simulink model "two_blocks_w_spring"  (R2017a)
settings: Solver=VariableStepAuto  StartTime=0.0  StopTime=40  RelTol=1e-3
values from neighbouring files (symbols this model uses):
  a = 20    [two_block_spring.mat]
  d_e = 0.5    [animation_two_block_spring.m]    (also in two_block_spring.mat)
  e_h = -1    [animation_two_block_spring.m]    (also in two_block_spring.mat = 1)
  e_v = -1    [animation_two_block_spring.m]    (also in two_block_spring.mat = 1)
  g = 9.81    [two_block_spring.mat]
  k = 5    [two_block_spring.mat]
  m_h = [-w_h w_h w_h -w_h -w_h ; w_h w_h -w_h -w_h w_h]    [animation_two_block_spring.m]    (also in two_block_spring.mat = 1)
  m_v = [-w_v w_v w_v -w_v -w_v ; w_v w_v -w_v -w_v w_v]    [animation_two_block_spring.m]    (also in two_block_spring.mat = 0.5)
  mu_h = 0.1    [two_block_spring.mat]
  mu_v = 0.2    [two_block_spring.mat]
settings Model: Creator=Sorawit Inprom  LastModifiedBy=Sorawit Inprom

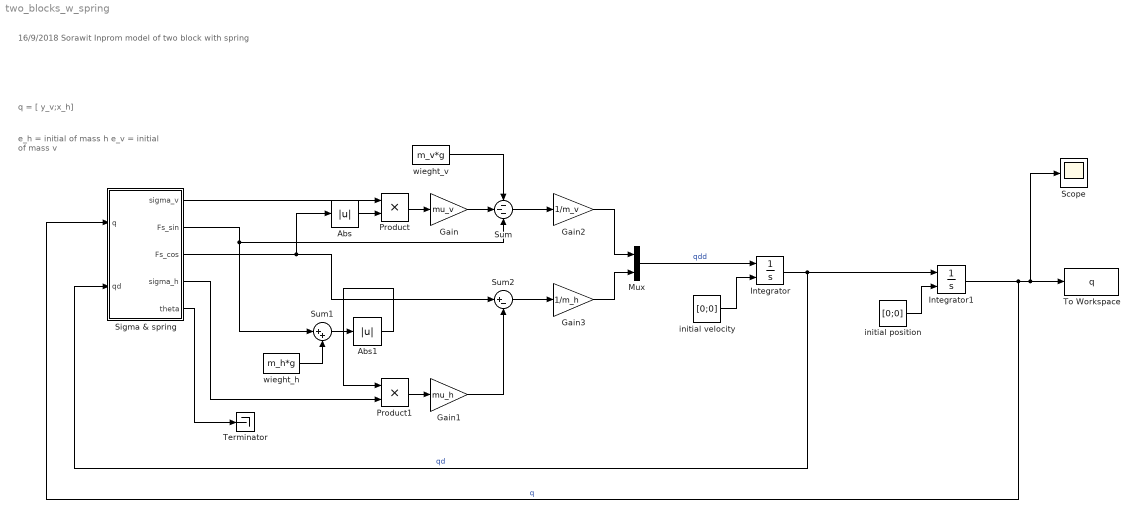
== system two_blocks_w_spring ==
  note: 16/9/2018
      | Sorawit Inprom
      | model of two block with spring
  note: e_h = initial of mass h
      | e_v = initial of mass v
  note: q = [ y_v;x_h]
  Abs : Abs
  Abs1 : Abs
  Gain : Gain  Gain=mu_v
  Gain1 : Gain  Gain=mu_h
  Gain2 : Gain  Gain=1/m_v
  Gain3 : Gain  Gain=1/m_h
  Integrator : Integrator  InitialConditionSource=external  InitialCondition=[0;0]  ContinuousStateAttributes='velocity'
  Integrator1 : Integrator  InitialConditionSource=external  InitialCondition=[e_v;e_h]  ContinuousStateAttributes='position'
  Mux : Mux  Inputs=2
  Product : Product
  Product1 : Product
  Scope : Scope
  Sigma & spring : Subsystem
  Sum : Sum  Inputs=---
  Sum1 : Sum  Inputs=|++
  Sum2 : Sum  Inputs=|+-
  Terminator : Terminator
  To Workspace : ToWorkspace  VariableName=q  SaveFormat=Timeseries  SampleTime=-1
  initial position : Constant  Value=[0;0]
  initial velocity : Constant  Value=[0;0]
  wieght_h : Constant  Value=m_h*g
  wieght_v : Constant  Value=m_v*g
  wires:
  Integrator/1 -> Sigma & spring/2(qd), Integrator1/1  "qd"
  Mux/1 -> Integrator/1  "qdd"
  wieght_v/1 -> Sum/1
  Product/1 -> Gain/1
  Product1/1 -> Gain1/1
  Gain1/1 -> Sum2/2
  Gain/1 -> Sum/2
  wieght_h/1 -> Sum1/2
  Sum/1 -> Gain2/1
  Sum2/1 -> Gain3/1
  Gain2/1 -> Mux/1
  Gain3/1 -> Mux/2
  initial velocity/1 -> Integrator/2
  initial position/1 -> Integrator1/2
  Integrator1/1 -> Sigma & spring/1(q), Scope/1, To Workspace/1  "q"
  Sigma & spring/1(sigma_v) -> Product/1
  Sigma & spring/3(Fs_cos) -> Abs/1, Sum2/1
  Sigma & spring/2(Fs_sin) -> Sum1/1, Sum/3
  Sigma & spring/4(sigma_h) -> Product1/2
  Sigma & spring/5("theta ") -> Terminator/1
  Abs/1 -> Product/2
  Sum1/1 -> Abs1/1
  Abs1/1 -> Product1/1

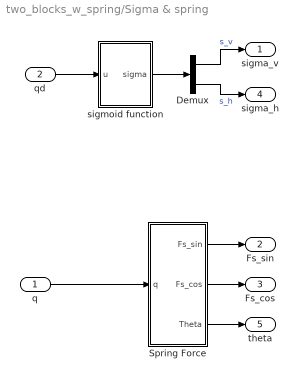
== system two_blocks_w_spring/Sigma & spring ==
  q : Inport
  qd : Inport  Port=2
  Demux : Demux  Outputs=2
  Spring Force : Subsystem
  sigmoid function : Subsystem
  sigma_v : Outport
  Fs_sin : Outport  Port=2
  Fs_cos : Outport  Port=3
  sigma_h : Outport  Port=4
  "theta " : Outport  Port=5
  wires:
  Demux/1 -> sigma_v/1  "s_v"
  q/1 -> Spring Force/1(q)
  sigmoid function/1(sigma) -> Demux/1
  Spring Force/1(Fs_sin) -> Fs_sin/1
  Spring Force/2(Fs_cos) -> Fs_cos/1
  qd/1 -> sigmoid function/1(u)
  Demux/2 -> sigma_h/1  "s_h"
  Spring Force/3(Theta) -> "theta "/1

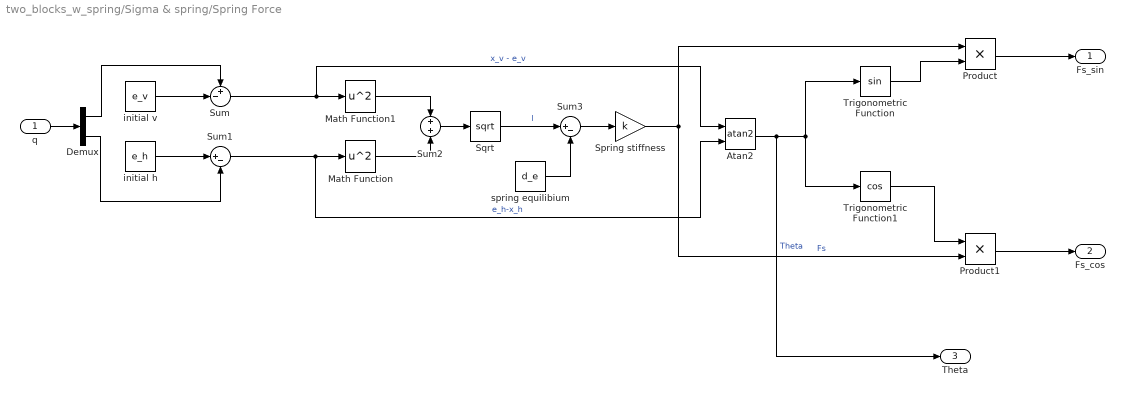
== system two_blocks_w_spring/Sigma & spring/Spring Force ==
  q : Inport
  Atan2 : Trigonometry  Operator=atan2
  Demux : Demux  Outputs=2
  Math Function : Math  Operator=square  SaturateOnIntegerOverflow=on
  Math Function1 : Math  Operator=square  SaturateOnIntegerOverflow=on
  Product : Product
  Product1 : Product
  Spring stiffness : Gain  Gain=k
  Sqrt : Sqrt  SaturateOnIntegerOverflow=on
  Sum : Sum  Inputs=+-|
  Sum1 : Sum  Inputs=|+-
  Sum2 : Sum  Inputs=+|+
  Sum3 : Sum  Inputs=|+-
  Trigonometric Function : Trigonometry
  Trigonometric Function1 : Trigonometry  Operator=cos
  initial h : Constant  Value=e_h
  initial v : Constant  Value=e_v
  spring equilibium : Constant  Value=d_e
  Fs_sin : Outport
  Fs_cos : Outport  Port=2
  Theta : Outport  Port=3
  wires:
  initial v/1 -> Sum/2
  Sqrt/1 -> Sum3/1  "l"
  Atan2/1 -> Theta/1, Trigonometric Function1/1, Trigonometric Function/1  "Theta"
  initial h/1 -> Sum1/1
  Sum1/1 -> Math Function/1, Atan2/2  "e_h-x_h"
  q/1 -> Demux/1
  Sum/1 -> Math Function1/1, Atan2/1  "x_v - e_v"
  Demux/1 -> Sum/1
  Demux/2 -> Sum1/2
  Math Function1/1 -> Sum2/1
  Math Function/1 -> Sum2/2
  Sum2/1 -> Sqrt/1
  spring equilibium/1 -> Sum3/2
  Sum3/1 -> Spring stiffness/1
  Spring stiffness/1 -> Product1/2, Product/1  "Fs"
  Trigonometric Function/1 -> Product/2
  Trigonometric Function1/1 -> Product1/1
  Product/1 -> Fs_sin/1
  Product1/1 -> Fs_cos/1

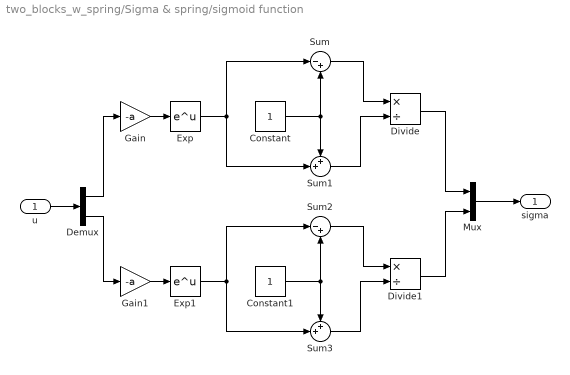
== system two_blocks_w_spring/Sigma & spring/sigmoid function ==
  u : Inport
  Constant : Constant
  Constant1 : Constant
  Demux : Demux  Outputs=2
  Divide : Product  Inputs=*/
  Divide1 : Product  Inputs=*/
  Exp : Math  SaturateOnIntegerOverflow=on
  Exp1 : Math  SaturateOnIntegerOverflow=on
  Gain : Gain  Gain=-a
  Gain1 : Gain  Gain=-a
  Mux : Mux  Inputs=2
  Sum : Sum  Inputs=|-+
  Sum1 : Sum  Inputs=++|
  Sum2 : Sum  Inputs=|-+
  Sum3 : Sum  Inputs=++|
  sigma : Outport
  wires:
  Sum1/1 -> Divide/2
  Gain/1 -> Exp/1
  Sum/1 -> Divide/1
  Exp/1 -> Sum1/2, Sum/1
  Constant/1 -> Sum1/1, Sum/2
  Constant1/1 -> Sum3/1, Sum2/2
  Exp1/1 -> Sum3/2, Sum2/1
  Sum2/1 -> Divide1/1
  Sum3/1 -> Divide1/2
  Gain1/1 -> Exp1/1
  u/1 -> Demux/1
  Demux/1 -> Gain/1
  Demux/2 -> Gain1/1
  Divide/1 -> Mux/1
  Divide1/1 -> Mux/2
  Mux/1 -> sigma/1
